simulink model "FirstOrderResponseForGlider"  (R2013a)
settings: Solver=ode3  StartTime=0.0  StopTime=30  FixedStep=1e-2  RelTol=1e-3
libraries: simulink x1
settings Model: Creator=user  LastModifiedBy=user

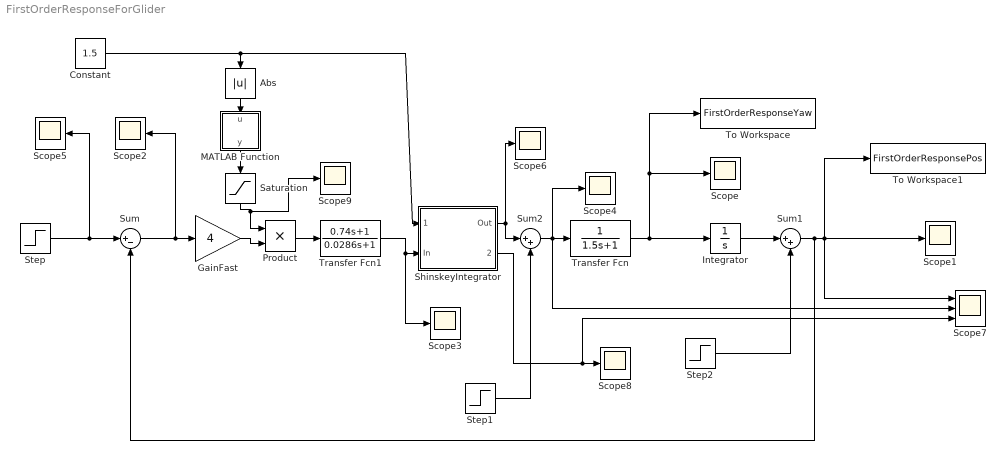
== system FirstOrderResponseForGlider ==
  Abs : Abs
  Constant : Constant  Value=1.5
  GainFast : Gain  Gain=4
  Integrator : Integrator
  MATLAB Function : MATLAB Function  TreatAsAtomicUnit=on
  Product : Product
  Saturation : Saturate  UpperLimit=1  LowerLimit=0.01
  Scope{,1..6,8..9} (9 alike) : Scope
      Scope1 settings: TimeRange=60  YMin=0  YMax=0.12
      Scope2 settings: SaveName=ScopeData2
      Scope3 settings: SaveName=ScopeData3
      Scope4 settings: SaveName=ScopeData4
      Scope5 settings: SaveName=ScopeData5
      Scope6 settings: SaveName=ScopeData6
      Scope8 settings: SaveName=ScopeData8
      Scope9 settings: SaveName=ScopeData9
  Scope7 : Scope  NumInputPorts=3
      settings: YMin=-5~-5~-1  YMax=5~5~2  SaveName=ScopeData7
  ShinskeyIntegrator : Subsystem
  Step : Step  Time=5  After=0.1  SampleTime=0
  Step1 : Step  Time=20  After=0.0  SampleTime=0
  Step2 : Step  Time=50  After=0  SampleTime=0
  Sum : Sum  Inputs=|+-
  Sum1 : Sum  Inputs=|++
  Sum2 : Sum  Inputs=|++
  To Workspace : ToWorkspace  VariableName=FirstOrderResponseYaw  SampleTime=-1
  To Workspace1 : ToWorkspace  VariableName=FirstOrderResponsePos  SampleTime=-1
  Transfer Fcn : TransferFcn  Denominator=[1.5 1]
  Transfer Fcn1 : TransferFcn  Numerator=[0.74 1]  Denominator=[0.0286 1]
  wires:
  Step/1 -> Scope5/1, Sum/1
  Transfer Fcn/1 -> Integrator/1, Scope/1, To Workspace/1
  Sum/1 -> Scope2/1, GainFast/1
  Integrator/1 -> Sum1/1
  GainFast/1 -> Product/2
  ShinskeyIntegrator/1(Out) -> Sum2/1, Scope6/1
  Transfer Fcn1/1 -> Scope3/1, ShinskeyIntegrator/2(In)
  Constant/1 -> Abs/1, ShinskeyIntegrator/1(BodyFixedVel)
  Sum1/1 -> To Workspace1/1, Scope7/1, Scope1/1, Sum/2
  Sum2/1 -> Scope7/2, Scope4/1, Transfer Fcn/1
  Step1/1 -> Sum2/2
  Step2/1 -> Sum1/2
  ShinskeyIntegrator/2(Saturated) -> Scope7/3, Scope8/1
  Saturation/1 -> Product/1, Scope9/1
  Product/1 -> Transfer Fcn1/1
  Abs/1 -> MATLAB Function/1(u)
  MATLAB Function/1(y) -> Saturation/1

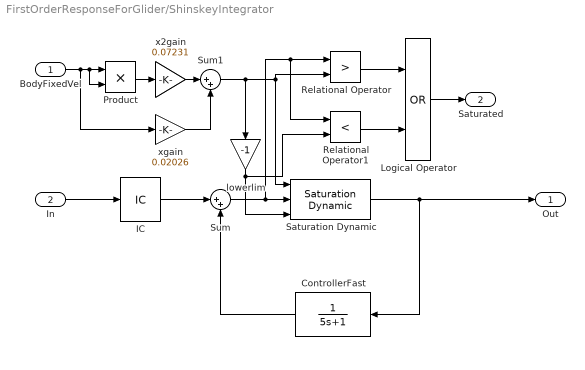
== system FirstOrderResponseForGlider/ShinskeyIntegrator ==
  BodyFixedVel : Inport
  In : Inport  Port=2
  ControllerFast : TransferFcn  Denominator=[5 1]
  IC : InitialCondition  Value=0
  Logical Operator : Logic  Operator=OR  AllPortsSameDT=off  OutDataTypeStr=boolean
  Product : Product
  Relational Operator : RelationalOperator  Operator=>  OutDataTypeStr=boolean
  Relational Operator1 : RelationalOperator  Operator=<  OutDataTypeStr=boolean
  Saturation Dynamic : simulink/Discontinuities/Saturation Dynamic  OutMin=[]  OutMax=[]  OutDataTypeStr=Inherit: Same as second input  OutDataType=fixdt(1, 16)  OutScaling=2^-10  DoSatur=off
  Sum : Sum  Inputs=|++
  Sum1 : Sum  Inputs=|++
  lowerlim : Gain  Gain=-1
  x2gain : Gain  Gain=0.07231
  xgain : Gain  Gain=0.02026
  Out : Outport
  Saturated : Outport  Port=2
  wires:
  In/1 -> IC/1
  Saturation Dynamic/1 -> ControllerFast/1, Out/1
  Sum/1 -> Relational Operator1/1, Relational Operator/1, Saturation Dynamic/2
  ControllerFast/1 -> Sum/2
  Sum1/1 -> Saturation Dynamic/1, Relational Operator/2, lowerlim/1
  lowerlim/1 -> Relational Operator1/2, Saturation Dynamic/3
  BodyFixedVel/1 -> xgain/1, Product/2, Product/1
  Product/1 -> x2gain/1
  x2gain/1 -> Sum1/1
  xgain/1 -> Sum1/2
  Relational Operator/1 -> Logical Operator/1
  Relational Operator1/1 -> Logical Operator/2
  Logical Operator/1 -> Saturated/1
  IC/1 -> Sum/1

== matlab function FirstOrderResponseForGlider/MATLAB Function ==
  data: u input; y output
function y = fcn(u)
%#codegen

y = u;
